simulink model "Trab1_desafio1"  (R2018a)
settings: Solver=VariableStepAuto  StartTime=0.0  StopTime=10.0  RelTol=1e-3
values from neighbouring files (symbols this model uses):
  A = [0 1 0 0; -K/M 0 K/M 0; 0 0 0 1; K/M 0 -K/M 0]    [Trab1_desafio_1.m]    (also in Trab1_desafio_2.m; Trabalho_1.m; calc_u.m = [0 1 0 0; -1.5 0 1.5 0; 0 0 0 1; 1.5 0 -1.5 0])
  B = [0 0; 1/M 0; 0 0; 0 1/M]    [Trab1_desafio_1.m]    (also in Trab1_desafio_2.m; Trabalho_1.m; calc_u.m = [0 0; 1.5 0; 0 0; 0 1.5])
  C = [1 0 0 0; 0 0 1 0]    [Trab1_desafio_1.m]    (also in Trab1_desafio_2.m; Trabalho_1.m)
  Tf = 5    [Trab1_desafio_1.m]    (also in Trab1_desafio_2.m; Trabalho_1.m)
settings Model: Creator=eric-  LastModifiedBy=eric-

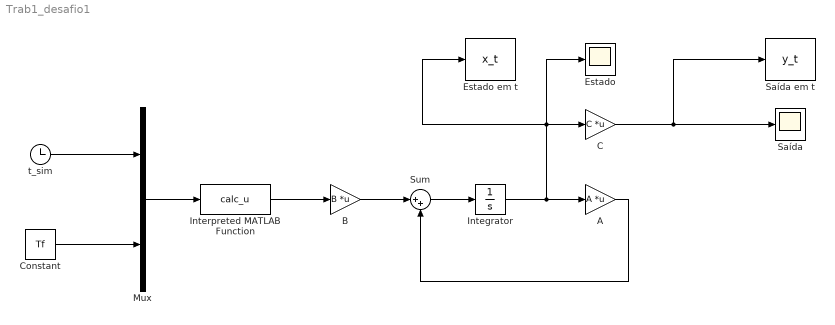
== system Trab1_desafio1 ==
  A : Gain  Gain=A  Multiplication=Matrix(K*u)
  B : Gain  Gain=B  Multiplication=Matrix(K*u)
  C : Gain  Gain=C  Multiplication=Matrix(K*u)
  Constant : Constant  Value=Tf
  "Estado " : Scope
  "Estado em t " : ToWorkspace  VariableName=x_t  SampleTime=-1
      settings: Save2DSignal=2-D array (concatenate along first dimension)
  Integrator : Integrator  InitialCondition=[5; 0; 5; 0]
  Interpreted MATLAB Function : MATLABFcn  MATLABFcn=calc_u  OutputDimensions=[2 1]  Output1D=off
  Mux : Mux  Inputs=2
  Saída : Scope
  Saída em t : ToWorkspace  VariableName=y_t  SampleTime=-1
      settings: Save2DSignal=2-D array (concatenate along first dimension)
  Sum : Sum  Inputs=|++
  "t_sim " : Clock
  wires:
  Sum/1 -> Integrator/1
  A/1 -> Sum/2
  B/1 -> Sum/1
  C/1 -> Saída/1, Saída em t/1
  Integrator/1 -> "Estado "/1, "Estado em t "/1, C/1, A/1
  "t_sim "/1 -> Mux/1
  Mux/1 -> Interpreted MATLAB Function/1
  Interpreted MATLAB Function/1 -> B/1
  Constant/1 -> Mux/2
